simulink model "FOSMCControllerCartPendulum"  (R2022b)
settings: Solver=ode14x  StartTime=0.0  StopTime=t_end  FixedStep=dt  RelTol=1e-3  EnableMultiTasking=on
values from neighbouring files (symbols this model uses):
  A = (M+m)*(J+m*L^2)    (= 0.0651)    [Basinofattraction.m]    (also in MainCEoptCase1_FOSMC.m; MainCEoptCase1_SMC.m; MainGAoptCase1_FOSMC.m; MainGAoptCase1_SMC.m)
  B = m*L    (= 0.05)    [Basinofattraction.m]    (also in MainCEoptCase1_FOSMC.m; MainCEoptCase1_SMC.m; MainGAoptCase1_FOSMC.m; MainGAoptCase1_SMC.m)
  C = M+m    (= 2.1)    [Basinofattraction.m]    (also in MainCEoptCase1_FOSMC.m; MainCEoptCase1_SMC.m; MainGAoptCase1_FOSMC.m; MainGAoptCase1_SMC.m)
  dtheta0 = 0.0*pi/180    (= 0)    [MainCEoptCase1_FOSMC.m]    (also in MainCEoptCase1_SMC.m; MainGAoptCase1_FOSMC.m; MainGAoptCase1_SMC.m)
  dxdisp0 = 0.0    (= 0)    [Basinofattraction.m]    (also in MainCEoptCase1_FOSMC.m; MainCEoptCase1_SMC.m; MainGAoptCase1_FOSMC.m; MainGAoptCase1_SMC.m)
  k = Xopt(1)    [Basinofattraction.m]    (also in MainCEoptCase1_FOSMC.m = x(1); MainCEoptCase1_SMC.m = x(1); MainGAoptCase1_FOSMC.m = x(1); MainGAoptCase1_SMC.m = x(1))
  lambda1 = Xopt(2)    [Basinofattraction.m]    (also in MainCEoptCase1_FOSMC.m = x(2); MainCEoptCase1_SMC.m = x(2); MainGAoptCase1_FOSMC.m = x(2); MainGAoptCase1_SMC.m = x(2))
  lambda2 = x(3)    [MainCEoptCase1_FOSMC.m]    (also in MainGAoptCase1_FOSMC.m)
  lambda3 = x(4)    [MainCEoptCase1_FOSMC.m]    (also in MainGAoptCase1_FOSMC.m)
  r = 0.0    (= 0)    [Basinofattraction.m]    (also in MainCEoptCase1_FOSMC.m; MainCEoptCase1_SMC.m; MainGAoptCase1_FOSMC.m; MainGAoptCase1_SMC.m)
  theta0 = theta0_deg * pi / 180    [Basinofattraction.m]    (also in MainCEoptCase1_FOSMC.m = 0.174532925199; MainCEoptCase1_SMC.m = 0.174532925199; MainGAoptCase1_FOSMC.m = 0.174532925199; MainGAoptCase1_SMC.m = 0.174532925199)
  xdisp0 = 0.0    (= 0)    [Basinofattraction.m]    (also in MainCEoptCase1_FOSMC.m; MainCEoptCase1_SMC.m; MainGAoptCase1_FOSMC.m; MainGAoptCase1_SMC.m)
libraries: fod x1
settings Model: Creator=julio  LastModifiedBy=Ana Cláudia Rubim
settings SolverCC: AlgebraicLoopSolver=TrustRegion
settings DataIOCC: ReturnWorkspaceOutputs=off
settings OptimizationCC: LifeSpan=inf
settings DebuggingCC: UnconnectedInputMsg=warning  UnconnectedOutputMsg=warning  UnconnectedLineMsg=warning  SFUnexpectedBacktrackingDiag=warning  SFNoUnconditionalDefaultTransitionDiag=warning  SFMachineParentedDataDiag=warning  ArithmeticOperatorsInVariantConditions=warning
settings ModelReferenceCC: EnableRefExpFcnMdlSchedulingChecks=on
settings SFSimCC: SimUseLocalCustomCode=off  CustomCodeUndefinedFunction=UseInterfaceOnly
settings RTWCC: RTWUseLocalCustomCode=off
settings CodeAppCC: StateflowObjectComments=on
settings GRTTargetCC: TargetLangStandard=C89/C90 (ANSI)
settings ConfigComp: CovMetricSettings=dw  CovSaveCumulativeToWorkspaceVar=on  CovSaveSingleToWorkspaceVar=on  CovExternalEMLEnable=off

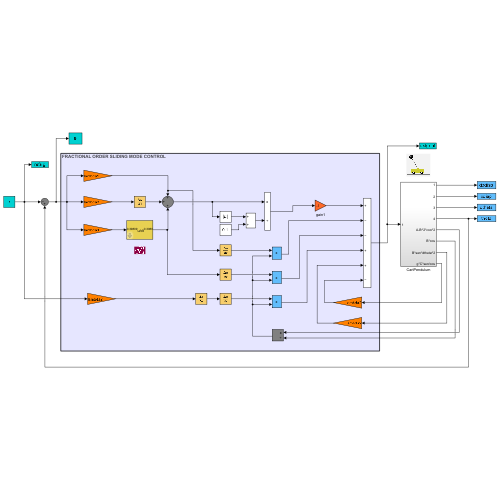
[thumbnail: Simulink's stored preview of the top-level diagram]
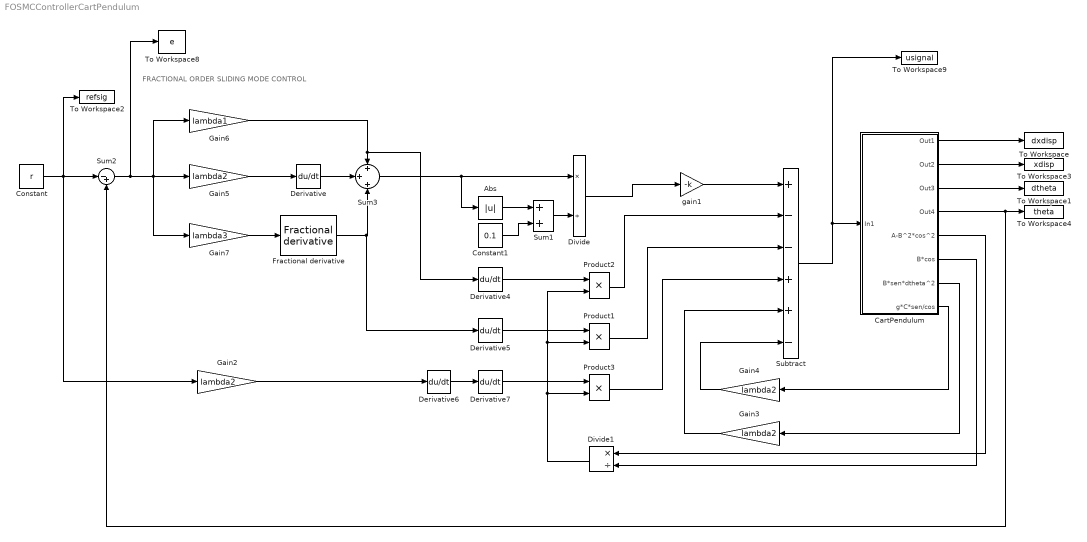
== system FOSMCControllerCartPendulum ==
  note: FRACTIONAL ORDER SLIDING MODE CONTROL
  Abs : Abs  ZeroCross=off  SaturateOnIntegerOverflow=off
  CartPendulum : Subsystem
  Constant : Constant  Value=r
  Constant1 : Constant  Value=0.1
  Derivative{,4..7} (5 alike) : Derivative
  Divide : Product  Inputs=*/
  Divide1 : Product  Inputs=*/
  Fractional derivative : fod/Fractional derivative  gam=OrderD  ww=[0.001; 1000]  n=5  nFod=off
      settings: SourceProductName=FOMCON Toolbox
  Gain{2..5} (4 alike) : Gain  Gain=lambda2
  Gain6 : Gain  Gain=lambda1
  Gain7 : Gain  Gain=lambda3
  Product1 : Product
  Product2 : Product
  Product3 : Product
  Subtract : Sum  Inputs=+--++-
  Sum1 : Sum
  Sum2 : Sum  Inputs=|-+
  Sum3 : Sum  Inputs=+|+|+
  To Workspace : ToWorkspace  VariableName=dxdisp  SampleTime=-1
  To Workspace1 : ToWorkspace  VariableName=dtheta  SampleTime=-1
  To Workspace2 : ToWorkspace  VariableName=refsig  SampleTime=-1
  To Workspace3 : ToWorkspace  VariableName=xdisp  SampleTime=-1
  To Workspace4 : ToWorkspace  VariableName=theta  SampleTime=-1
  To Workspace8 : ToWorkspace  VariableName=e  SampleTime=-1
  To Workspace9 : ToWorkspace  VariableName=usignal  SampleTime=-1
  gain1 : Gain  Gain=-k
  wires:
  Subtract/1 -> To Workspace9/1, CartPendulum/1(In1)
  Gain5/1 -> Derivative/1
  Gain6/1 -> Derivative4/1, Sum3/1
  Derivative/1 -> Sum3/2
  Gain7/1 -> Fractional derivative/1
  Fractional derivative/1 -> Derivative5/1, Sum3/3
  Sum2/1 -> To Workspace8/1, Gain7/1, Gain6/1, Gain5/1
  CartPendulum/2(Out2) -> To Workspace3/1
  CartPendulum/3(Out3) -> To Workspace1/1
  CartPendulum/4(Out4) -> Sum2/2, To Workspace4/1
  CartPendulum/1(Out1) -> To Workspace/1
  Constant/1 -> Gain2/1, To Workspace2/1, Sum2/1
  Constant1/1 -> Sum1/2
  Sum1/1 -> Divide/2
  gain1/1 -> Subtract/1
  Sum3/1 -> Abs/1, Divide/1
  Abs/1 -> Sum1/1
  CartPendulum/8(g*C*sen/cos) -> Gain4/1
  CartPendulum/7(B*sen*dtheta^2) -> Gain3/1
  CartPendulum/5(A-B^2*cos^2) -> Divide1/1
  CartPendulum/6(B*cos) -> Divide1/2
  Derivative6/1 -> Derivative7/1
  Derivative4/1 -> Product2/1
  Derivative5/1 -> Product1/1
  Derivative7/1 -> Product3/1
  Divide1/1 -> Product2/2, Product1/2, Product3/2
  Product2/1 -> Subtract/2
  Product1/1 -> Subtract/3
  Product3/1 -> Subtract/4
  Gain2/1 -> Derivative6/1
  Gain3/1 -> Subtract/5
  Gain4/1 -> Subtract/6
  Divide/1 -> gain1/1

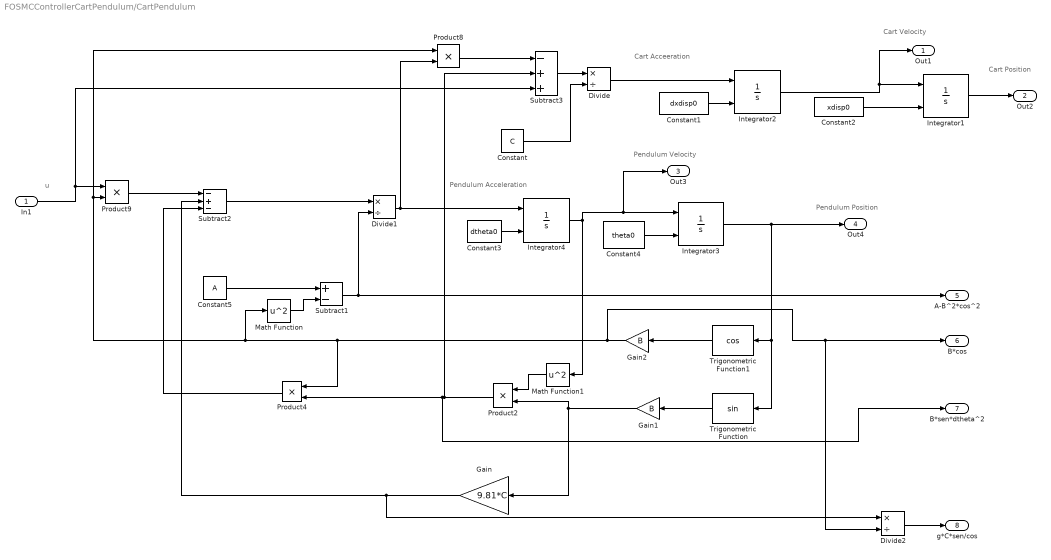
== system FOSMCControllerCartPendulum/CartPendulum ==
  note: u
  note: Pendulum Acceleration
  note: Pendulum Position
  note: Cart Acceeration
  note: Cart Velocity
  note: Cart Position
  note: Pendulum Velocity
  In1 : Inport
  Constant : Constant  Value=C
  Constant1 : Constant  Value=dxdisp0
  Constant2 : Constant  Value=xdisp0
  Constant3 : Constant  Value=dtheta0
  Constant4 : Constant  Value=theta0
  Constant5 : Constant  Value=A
  Divide : Product  Inputs=*/
  Divide1 : Product  Inputs=*/
  Divide2 : Product  Inputs=*/
  Gain : Gain  Gain=9.81*C
  Gain1 : Gain  Gain=B
  Gain2 : Gain  Gain=B
  Integrator{1..4} (4 alike) : Integrator  InitialConditionSource=external
  Math Function : Math  Operator=square  SignedPower=on
  Math Function1 : Math  Operator=square  SignedPower=on
  Product{2,4,8..9} (4 alike) : Product
  Subtract1 : Sum  Inputs=+-
  Subtract2 : Sum  Inputs=-+-
  Subtract3 : Sum  Inputs=-++
  Trigonometric Function : Trigonometry
  Trigonometric Function1 : Trigonometry  Operator=cos
  Out1 : Outport
  Out2 : Outport  Port=2
  Out3 : Outport  Port=3
  Out4 : Outport  Port=4
  A-B^2*cos^2 : Outport  Port=5
  B*cos : Outport  Port=6
  B*sen*dtheta^2 : Outport  Port=7
  g*C*sen/cos : Outport  Port=8
  wires:
  Integrator4/1 -> Math Function1/1, Out3/1, Integrator3/1
  Gain2/1 -> Divide2/2, B*cos/1, Product4/1, Math Function/1, Product8/1, Product9/2
  Product9/1 -> Subtract2/1
  Constant2/1 -> Integrator1/2
  Subtract2/1 -> Divide1/1
  Integrator2/1 -> Out1/1, Integrator1/1
  Divide/1 -> Integrator2/1
  Trigonometric Function1/1 -> Gain2/1
  Subtract1/1 -> Divide1/2, A-B^2*cos^2/1
  Divide1/1 -> Integrator4/1, Product8/2
  Math Function/1 -> Subtract1/2
  Math Function1/1 -> Product2/1
  Gain1/1 -> Gain/1, Product2/2
  Product8/1 -> Subtract3/1
  Subtract3/1 -> Divide/1
  Product4/1 -> Subtract2/3
  Product2/1 -> Subtract3/2, B*sen*dtheta^2/1, Product4/2
  In1/1 -> Subtract3/3, Product9/1
  Gain/1 -> Divide2/1, Subtract2/2
  Constant/1 -> Divide/2
  Integrator3/1 -> Out4/1, Trigonometric Function/1, Trigonometric Function1/1
  Constant4/1 -> Integrator3/2
  Constant3/1 -> Integrator4/2
  Constant1/1 -> Integrator2/2
  Constant5/1 -> Subtract1/1
  Trigonometric Function/1 -> Gain1/1
  Integrator1/1 -> Out2/1
  Divide2/1 -> g*C*sen/cos/1
